simulink library "DABLib"  (R2016b)
settings: Solver=VariableStepAuto  StartTime=0.0  StopTime=10.0  RelTol=1e-3
undefined symbols (not defined in the file or in its folder): ln, sgn
libraries: DABLib x53, simulink_extras x2, simulink x1
(part 1 of 3)
settings Model: Creator=davidlaredorazo  LastModifiedBy=davidlaredorazo
settings DataIOCC: SaveFormat=Array  SignalLoggingSaveFormat=ModelDataLogs
settings OptimizationCC: BlockReduction=off  BooleanDataType=off
settings DebuggingCC: SaveWithParameterizedLinksMsg=none  UnderspecifiedInitializationDetection=Classic  MergeDetectMultiDrivingBlocksExec=none  SignalResolutionControl=TryResolveAllWithWarning  MultiTaskDSMMsg=warning  MultiTaskCondExecSysMsg=none  StrictBusMsg=None
settings HardwareCC: TargetUnknown=on
settings ModelReferenceCC: PropagateSignalLabelsOutOfModel=off

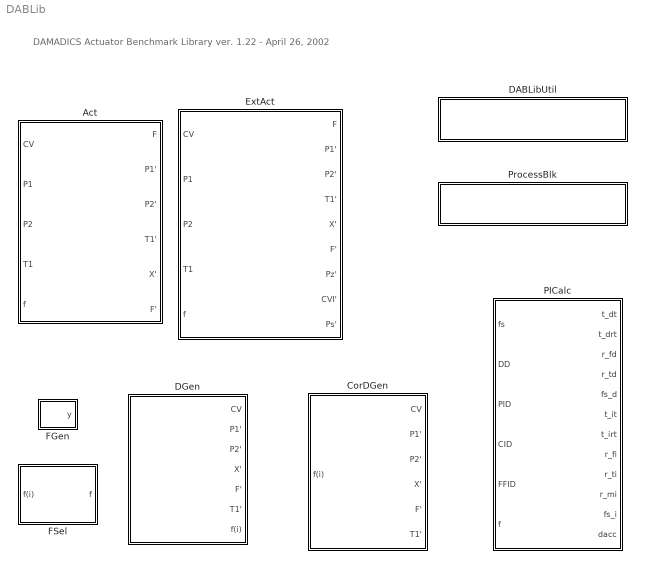
== system DABLib ==
  note: DAMADICS Actuator Benchmark Library ver. 1.22 - April 26, 2002
  Act : Subsystem  mask(Actuator){Dist=off}
      mask prompts: Dist "Disable noise"
      mask help:
      | Actuator 'Act' block is a core of a 'DABLib' library. This block is a model of final control element consisting of positioner, pneumatic motor, control valve and bypass valve.
      | This block reflects the virtual actuator however the parameters of the model were tuned using experimental data achieved during the laboratory tests of: positioner A785, servo-motor type 37 and equalpercentage control valve installed in steam boiler control loop.
      mask Help: web( [ 'file:///' which('DABLib.pdf')]);
      mask Display:
      | plot( [0.2 0.45], [0.3 0.3] )
      | plot( [0.75 0.8], [0.3 0.3] )
      | plot( [0.75 0.75 0.45 0.45 0.75], [0.1 0.5 0.1 0.5 0.1] )
      | plot( [0.6 0.6], [0.3 0.6])
      | plot( [0.45 0.75 0.70 0.5 0.45], [0.6 0.6 0.7 0.7 0.6] )
      | plot( [0.25 0.35 0.35 0.45], [0.9 0.7 0.75 0.55] )
      | text(0.4, 0.9, 'f')
  CorDGen : Subsystem  mask(Benchmark data generator){FSel=NO FAULT}
      mask prompts: FSel "Fault selector:"
      mask help: Data generator 'HIDGen' is a block allowing the generation of data sets with hidden faults for benchmark purposes.
      mask Help: web( [ 'file:///' which('DABLib.pdf')]);
      mask TypeOptions FSel: f1 - Valve clogging | f2 - Valve plug or valve seat sedimentation | f3 - Valve plug or valve seat erosion | f4 - Increased of valve or bushing friction | f5 - External leakage | f6 - Internal leakage | f7 - Medium evaporation or critical flow | f8 - Twisted servo-motor's piston rod | f9 - Servo-motor's housing or terminals tightness | f10 - Servo-motor's diaphragm perforation | f11 - Servo-motor's spring fault | f12 - Electro-pneumatic transducer fault | f13 - Rod displacement sensor fault | f14 - Pressure sensor fault | f15 - Positioner feedback fault | f16 - Positioner supply pressure drop | f17 - Unexpected pressure change across the valve | f18 - Fully or partly opened bypass valves | f19 - Flow rate sensor fault | NO FAULT
      mask Display: fprintf( 'Benchmark Data\n with Hidden Fault\n Generator' )
  DABLibUtil : Subsystem
      mask Display: fprintf(['DABLib Utilities'])
  DGen : Subsystem  mask(Benchmark data generator){FSel=NO FAULT, FType=Abrupt - Small}
      mask prompts: FSel "Fault selector:"; FType "Failure mode:"
      mask help:
      | Data generator 'DGen'  is a block allowing the generation of repeatable patterns of data sets for benchmark purposes.
      |
      | Attention!
      | Not all combinations of parameters are allowed for benchmark. In the case of wrong selection the simulation will be stopped.
      mask init:
      | DSim=0;
      | FSD=1;
      | FFrom = 900;
      | FTo = inf;
      | if FType==4
      |     FMFS=1;
      |     switch FSel
      |         case {2, 3, 5, 6, 9, 11, 18}
      |             FFDT = 3600*24;
      |         case {4, 17}
      |             FFDT = 3600;
      |         case {13}
      |             FFDT = 60*15;
      |         case {20}
      |             FFDT = 0;
      |         otherwise,
      |             FSel = 20;
      |             FFDT = 0;
      |             DSim=1;
      |             warning('Error! - Fault with selected type not specified for benchmark purpose.')
      |     end
      | else
      |     FMFS=0.25*FType;
      |     FFDT=0;
      |     switch FSel
      |         case {3, 4, 5, 6, 9}
      |             DSim=1;
      |             warning('Error! - Fault with selected type not specified for benchmark purpose.')
      |         case {2, 11, 15, 17}
      |             if FType<3
      |                 DSim=1;
      |                 warning('Error! - Fault with selected type not specified for benchmark purpose.')
      |             end
      |         otherwise,
      |     end
      | end
      | switch FSel
      |     case {12, 14, 19}
      |         FSD = -1;
      |     otherwise,
      | end
      mask Help: web( [ 'file:///' which('DABLib.pdf')]);
      mask TypeOptions FSel: f1 - Valve clogging | f2 - Valve plug or valve seat sedimentation | f3 - Valve plug or valve seat erosion | f4 - Increased of valve or bushing friction | f5 - External leakage | f6 - Internal leakage | f7 - Medium evaporation or critical flow | f8 - Twisted servo-motor's piston rod | f9 - Servo-motor's housing or terminals tightness | f10 - Servo-motor's diaphragm perforation | f11 - Servo-motor's spring fault | f12 - Electro-pneumatic transducer fault | f13 - Rod displacement sensor fault | f14 - Pressure sensor fault | f15 - Positioner feedback fault | f16 - Positioner supply pressure drop | f17 - Unexpected pressure change across the valve | f18 - Fully or partly opened bypass valves | f19 - Flow rate sensor fault | NO FAULT
      mask TypeOptions FType: Abrupt - Small | Abrupt - Medium | Abrupt - Large | Incipient
      mask Display: fprintf( 'Benchmark \n Data Generator' )
  ExtAct : Subsystem  mask(Extended Actuator){Dist=on}
      mask prompts: Dist "Disable noise / Analog Transmission"
      mask help:
      | This block is a model of final control element consisting of positioner, pneumatic motor, control valve and bypass valve.
      | This block reflects the virtual actuator however the parameters of the model were tuned using experimental data achieved during the laboratory tests of: positioner A785, servo-motor type 37 and equalpercentage control valve installed in steam boiler control loop.
      mask Help: web( [ 'file:///' which('DABLib.pdf')]);
      mask Display:
      | plot( [0.2 0.45], [0.3 0.3] )
      | plot( [0.75 0.8], [0.3 0.3] )
      | plot( [0.75 0.75 0.45 0.45 0.75], [0.1 0.5 0.1 0.5 0.1] )
      | plot( [0.6 0.6], [0.3 0.6])
      | plot( [0.45 0.75 0.70 0.5 0.45], [0.6 0.6 0.7 0.7 0.6] )
      | plot( [0.25 0.35 0.35 0.45], [0.85 0.7 0.75 0.55] )
      | text(0.4, 0.9, 'f')
      | text(0.2, 1.05, '<<< Extended >>>')
      | text(0.01, 0.03, 'Only for extended researches')
  FGen : Subsystem  mask(Fault generator){From=300, To=inf, MFS=0.5, FDT=0, FSD=1}
      mask prompts: MFS "Max Fault Strength:"; FDT "Fault Development Time:"; FSD "Direction:"
      mask help:
      | Used for generation of abrupt and incipient standarised fault strength values.
      |
      | Parameters:
      | From - fault start time [s]
      | To - fault decay time [s]
      | Max Fault Strength - maximum fault strength value that will be reached during simulation [standarised range - 0 1]
      | Fault Development Time - after this time Max Fault Strength will be reached [s]
      | Direction - defines the sign of fault strength.
      mask init:
      | if FDT==0
      |  FDS = 99999999999999999999999999;
      | else
      |  FDS = MFS / FDT;
      | end
      | if To==inf
      |  To = 99999999999999999999999999;
      | end
      | if FSD >= 0
      | FSD=1;
      | else
      | FSD=-1;
      | end
      mask Help: web( [ 'file:///' which('DABLib.pdf')]);
      mask Display: disp('FGen')
  FSel : Subsystem  mask(Fault vector element attribution){FSel=NO FAULT}
      mask prompts: FSel "Fault selector"
      mask help:
      | Attributes input value to i-th element of the output fault strength vector. The size of the fault strength vector is 19. The values of other output vector elements are set to 0.
      | If 'NO FAULT' option is selected than the fault vector with all 0 elements is produced.
      mask Help: web( [ 'file:///' which('DABLib.pdf')]);
      mask TypeOptions FSel: f1 - Valve clogging | f2 - Valve plug or valve seat sedimentation | f3 - Valve plug or valve seat erosion | f4 - Increased of valve or bushing friction | f5 - External leakage | f6 - Internal leakage | f7 - Medium evaporation or critical flow | f8 - Twisted servo-motor's piston rod | f9 - Servo-motor's housing or terminals tightness | f10 - Servo-motor's diaphragm perforation | f11 - Servo-motor's spring fault | f12 - Electro-pneumatic transducer fault | f13 - Rod displacement sensor fault | f14 - Pressure sensor fault | f15 - Positioner feedback fault | f16 - Positioner supply pressure drop | f17 - Unexpected pressure change across the valve | f18 - Fully or partly opened bypass valves | f19 - Flow rate sensor fault | NO FAULT
      mask Display:
      | text(0.5, 0.75, 'f(i)')
      | plot( [0.5 0.5], [0.7 0.3] )
      | plot( [0.45 0.5 0.55], [0.4 0.3 0.4])
      | text(0.35, 0.1, '[ f(i)   ]')
  PICalc : Subsystem  mask(Performance Indexes Calculator){Step=Other, FSel=NO FAULT, FType=Abrupt - Small, t_on_ini=0, t_hor_ini=100}
      mask prompts: Step "Benchmark:"; FSel "Fault selector:"; FType "Failure mode:"; t_on_ini "Start of Benchmark Zone:"; t_hor_ini "End of Benchmark Zone:"
      mask init:
      | DSim = 0;
      | switch Step
      | 	case {1}
      |       t_on = 300;
      |       if FType==4
      |     		switch FSel
      |         		case {2, 3, 5, 6, 9, 11, 18}
      |             	t_hor = 85500;
      |         		case {4, 17}
      |             	t_hor = 5100;
      |         		case {13}
      |             	t_hor = 2400;
      |         		otherwise,
      |             	t_on = 0;
      |             	t_hor = 0;
      | 					DSim = 1;
      |             	warning('Error! - Fault with selected type not specified for benchmark purpose.')
      |     		end
      | 		else
      | 			t_hor = 1500;
      | 			switch FSel
      |         		case {3, 4, 5, 6, 9}
      |             	t_on = 0;
      |             	t_hor = 0;
      | 					DSim = 1;
      |             	warning('Error! - Fault with selected type not specified for benchmark purpose.')
      |         		case {2, 11, 15, 17}
      |             	if FType<3
      | 	            	t_on = 0;
      |    	         	t_hor = 0;
      | 						DSim = 1;
      |                   warning('Error! - Fault with selected type not specified for benchmark purpose.')
      |                end
      |         		otherwise,
      |     		end
      |       end
      |    case {2}
      | 	            	t_on = 0;
      |    	         	t_hor = 0;
      | 						DSim = 1;
      |                   warning('Not done yet!')
      | 	case {3}
      | 	            	t_on = 0;
      |    	         	t_hor = 0;
      | 						DSim = 1;
      |                   warning('Not done yet!')
      |    otherwise,
      |       t_on = t_on_ini;
      |       t_hor = t_hor_ini;
      | end
      mask TypeOptions Step: I Step | II Step | III Step | Other
      mask TypeOptions FSel: f1 - Valve clogging | f2 - Valve plug or valve seat sedimentation | f3 - Valve plug or valve seat erosion | f4 - Increased of valve or bushing friction | f5 - External leakage | f6 - Internal leakage | f7 - Medium evaporation or critical flow | f8 - Twisted servo-motor's piston rod | f9 - Servo-motor's housing or terminals tightness | f10 - Servo-motor's diaphragm perforation | f11 - Servo-motor's spring fault | f12 - Electro-pneumatic transducer fault | f13 - Rod displacement sensor fault | f14 - Pressure sensor fault | f15 - Positioner feedback fault | f16 - Positioner supply pressure drop | f17 - Unexpected pressure change across the valve | f18 - Fully or partly opened bypass valves | f19 - Flow rate sensor fault | NO FAULT
      mask TypeOptions FType: Abrupt - Small | Abrupt - Medium | Abrupt - Large | Incipient
      mask Display: fprintf( 'Performance\n Indexes\n Calculator' )
  ProcessBlk : Subsystem
      mask Display: fprintf(['Process Components'])

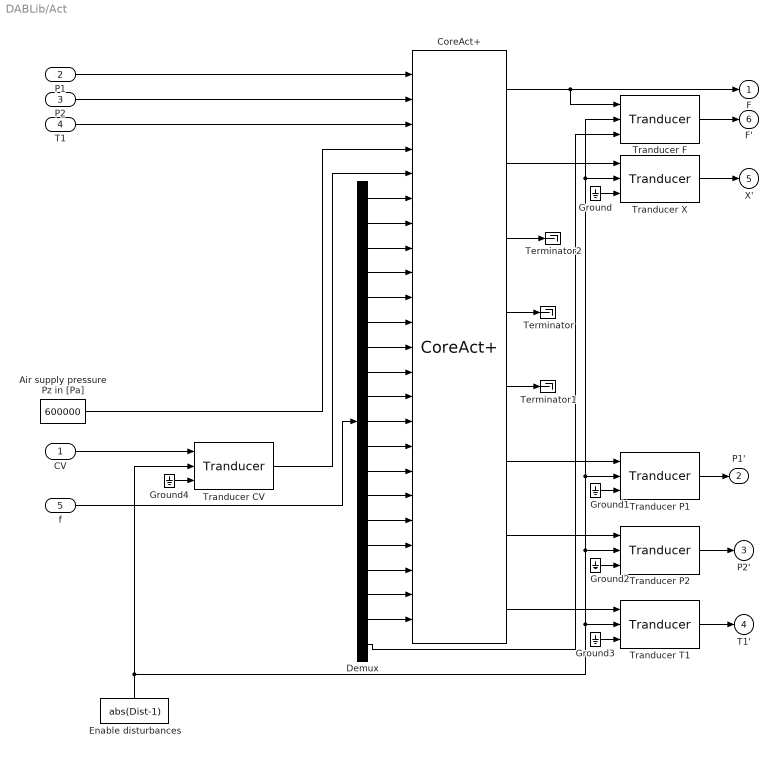
== system DABLib/Act ==
  CV : Inport
  P1 : Inport  Port=2
  P2 : Inport  Port=3
  T1 : Inport  Port=4
  f : Inport  Port=5
  Air supply pressure Pz in [Pa] : Constant  Value=600000
  CoreAct+ : DABLib/DABLibUtil/CoreAct+
  Demux : Demux  Outputs=19
  Enable disturbances : Constant  Value=abs(Dist-1)
  Ground{,1..4} (5 alike) : Ground
  Terminator : Terminator
  Terminator1 : Terminator
  Terminator2 : Terminator
  Tranducer CV : DABLib/DABLibUtil/Tranducer  ScFact=1  Sd=[435435431]
  Tranducer F : DABLib/DABLibUtil/Tranducer  ScFact=40  Sd=[324125]
  Tranducer P1 : DABLib/DABLibUtil/Tranducer  ScFact=4000000  Sd=[123465]
  Tranducer P2 : DABLib/DABLibUtil/Tranducer  ScFact=4000000  Sd=[143534565]
  Tranducer T1 : DABLib/DABLibUtil/Tranducer  ScFact=200  Sd=[452543]
  Tranducer X : DABLib/DABLibUtil/Tranducer  ScFact=1  Sd=[43543513]
  F : Outport  InitialOutput=0
  P1' : Outport  Port=2  InitialOutput=0
  P2' : Outport  Port=3  InitialOutput=0
  T1' : Outport  Port=4  InitialOutput=0
  X' : Outport  Port=5  InitialOutput=0
  F' : Outport  Port=6  InitialOutput=0
  wires:
  CoreAct+/3 -> Terminator2/1
  CoreAct+/4 -> Terminator/1
  CoreAct+/5 -> Terminator1/1
  CoreAct+/1 -> F/1, Tranducer F/1
  f/1 -> Demux/1
  CV/1 -> Tranducer CV/1
  Tranducer CV/1 -> CoreAct+/5
  Demux/1 -> CoreAct+/6
  Demux/2 -> CoreAct+/7
  Demux/3 -> CoreAct+/8
  Demux/4 -> CoreAct+/9
  Demux/5 -> CoreAct+/10
  Demux/6 -> CoreAct+/11
  Demux/7 -> CoreAct+/12
  Demux/8 -> CoreAct+/13
  Demux/9 -> CoreAct+/14
  Demux/10 -> CoreAct+/15
  Demux/11 -> CoreAct+/16
  Demux/12 -> CoreAct+/17
  Demux/13 -> CoreAct+/18
  Demux/14 -> CoreAct+/19
  Demux/15 -> CoreAct+/20
  Demux/16 -> CoreAct+/21
  Demux/17 -> CoreAct+/22
  Demux/18 -> CoreAct+/23
  Enable disturbances/1 -> Tranducer P1/2, Tranducer F/2, Tranducer X/2, Tranducer T1/2, Tranducer P2/2, Tranducer CV/2
  Air supply pressure Pz in [Pa]/1 -> CoreAct+/4
  P1/1 -> CoreAct+/1
  P2/1 -> CoreAct+/2
  Ground4/1 -> Tranducer CV/3
  T1/1 -> CoreAct+/3
  CoreAct+/2 -> Tranducer X/1
  Demux/19 -> Tranducer F/3
  Tranducer X/1 -> X'/1
  Tranducer F/1 -> F'/1
  CoreAct+/6 -> Tranducer P1/1
  Tranducer P1/1 -> P1'/1
  Ground1/1 -> Tranducer P1/3
  CoreAct+/7 -> Tranducer P2/1
  Tranducer P2/1 -> P2'/1
  Ground2/1 -> Tranducer P2/3
  Ground3/1 -> Tranducer T1/3
  Tranducer T1/1 -> T1'/1
  CoreAct+/8 -> Tranducer T1/1
  Ground/1 -> Tranducer X/3

== system DABLib/CorDGen ==
  f(i) : Inport
  Act : DABLib/Act  Dist=off
  Demux : Demux  Outputs=7
  FSel : DABLib/FSel  FSel=NO FAULT
  F_CV3 : Subsystem  mask(Sinus generator){A=0.25, f=0.01, c=0.5}
      mask prompts: A "Amplitude:"; f "Frequency:"; c "Constant component:"
      mask help: y= Asin( 2*3.14ft ) + const
      mask Help: web( [ 'file:///' which('wutalib.html')]);
      mask Display: disp('Sin-gen')
  F_CV4 : Subsystem  mask(Sinus generator){A=175000, f=0.1, c=3500000}
      mask prompts: A "Amplitude:"; f "Frequency:"; c "Constant component:"
      mask help: y= Asin( 2*3.14ft ) + const
      mask Help: web( [ 'file:///' which('wutalib.html')]);
      mask Display: disp('Sin-gen')
  F_CV5 : Subsystem  mask(Sinus generator){A=26000, f=1/pi, c=2600000}
      mask prompts: A "Amplitude:"; f "Frequency:"; c "Constant component:"
      mask help: y= Asin( 2*3.14ft ) + const
      mask Help: web( [ 'file:///' which('wutalib.html')]);
      mask Display: disp('Sin-gen')
  Mux1 : Mux  Inputs=7
  Terminator : Terminator
  "Water temperature [C] " : Constant  Value=43
  Zero-Order Hold : ZeroOrderHold
  CV : Outport  InitialOutput=0
  P1' : Outport  Port=2  InitialOutput=0
  P2' : Outport  Port=3  InitialOutput=0
  X' : Outport  Port=4  InitialOutput=0
  F' : Outport  Port=5  InitialOutput=0
  T1' : Outport  Port=6  InitialOutput=0
  wires:
  "Water temperature [C] "/1 -> Act/4
  FSel/1 -> Act/5
  Act/2 -> Mux1/3
  Act/3 -> Mux1/4
  Act/4 -> Mux1/5
  Act/5 -> Mux1/6
  Act/6 -> Mux1/7
  F_CV3/1(y) -> Act/1, Mux1/1
  Demux/1 -> CV/1
  Demux/2 -> Terminator/1
  Demux/3 -> P1'/1
  Demux/4 -> P2'/1
  Demux/5 -> T1'/1
  Demux/6 -> X'/1
  Demux/7 -> F'/1
  F_CV5/1(y) -> Act/3
  Mux1/1 -> Zero-Order Hold/1
  Zero-Order Hold/1 -> Demux/1
  F_CV4/1(y) -> Act/2
  Act/1 -> Mux1/2
  f(i)/1 -> FSel/1

== system DABLib/DABLibUtil ==
  -1 Correction : Subsystem
  0 Proof Division with -1 correction : Subsystem
  "0, t-t1>0, t2 or 0" : Subsystem
  ADist : Subsystem  mask(Artificial Disturbances){Sine=on, BLWN=on, Seed=[3525342532], ST=0.0025}
      mask prompts: Sine "Sine Enable:"; BLWN "BLWN Enable:"; ST "Sampling Time:"
      mask help: This block introduces artificial generated noise - disturbance.
      mask Help: web( [ 'file:///' which('DABLin.pdf')]);
      mask Display:
      | plot( [0.25 0.5 0.5], [0.25 0.25 0.65] )
      | plot( [0.45 0.5 0.55], [0.6 0.65 0.6])
      | plot( [0.25 0.5 0.51 0.55 0.59 0.61 0.65 0.68 0.7 0.75 0.78 0.8], [0.75 0.75 0.78 0.73 0.8 0.62 0.79 0.6 0.85 0.70 0.8 0.6] )
  ByVal : Subsystem  mask(Valve){}
      mask help: Internal library bloks - not for common use !!
      mask Help: web( [ 'file:///' which('DABLib.pdf')]);
      mask Display: fprintf( 'Bypass \n Valve' )
  Bypass valve opened or bypass valve leaky f18 : Subsystem
  CoreAct : Subsystem  mask(Actuator){}
      mask help: Internal library bloks - not for common use !!
      mask Help: web( [ 'file:///' which('DABLib.pdf')]);
      mask Display: fprintf( 'Core \n Actuator' )
  CoreAct+ : Subsystem  mask(Actuator){}
      mask help: Internal library bloks - not for common use !!
      mask Help: web( [ 'file:///' which('DABLib.pdf')]);
      mask Display: fprintf( 'Core \n Actuator \n + \n Bypass \n Valve \n + \n Ext. Faults' )
  Det or Iso : Subsystem
  Medium evaporation fault f7 : Subsystem
  "Medium evaporation fault f7 " : DABLib/DABLibUtil/Medium evaporation fault f7
  NFSel : Subsystem  mask(Fault vector element selection){FSel=NO FAULT}
      mask prompts: FSel "Fault selector"
      mask help:
      | Attributes i-th element of the input fault strength vector to output value. The size of the fault strength vector is 19.
      | If 'NO FAULT' option is selected than the 0 value is produced.
      mask Help: web( [ 'file:///' which('DABLib.pdf')]);
      mask TypeOptions FSel: f1 - Valve clogging | f2 - Valve plug or valve seat sedimentation | f3 - Valve plug or valve seat erosion | f4 - Increased of valve or bushing friction | f5 - External leakage | f6 - Internal leakage | f7 - Medium evaporation or critical flow | f8 - Twisted servo-motor's piston rod | f9 - Servo-motor's housing or terminals tightness | f10 - Servo-motor's diaphragm perforation | f11 - Servo-motor's spring fault | f12 - Electro-pneumatic transducer fault | f13 - Rod displacement sensor fault | f14 - Pressure sensor fault | f15 - Positioner feedback fault | f16 - Positioner supply pressure drop | f17 - Unexpected pressure change across the valve | f18 - Fully or partly opened bypass valves | f19 - Flow rate sensor fault | NO FAULT
      mask Display:
      | text(0.5, 0.1, 'f(i)')
      | plot( [0.5 0.5], [0.7 0.3] )
      | plot( [0.45 0.5 0.55], [0.4 0.3 0.4])
      | text(0.35, 0.75, '[ f(i)   ]')
  Positioner pressure supply fault f16 : Subsystem
  Tranducer : Subsystem  mask(Sensor){ScFact=1, Sd=[546547567568]}
      mask prompts: ScFact "Scalling Factor:"; Sd "Seed:"
  Treshold2 : Subsystem  mask(Decimal to Binary Conversion){TH=0.5}
      mask prompts: TH "Threshold:"
      mask Display: fprintf( 'Dec \n 2 \n Bin' )

== system DABLib/DGen ==
  Act : DABLib/Act  Dist=off
  Demux : Demux  Outputs=7
  Disable simulation : Constant  Value=DSim
  FGen : DABLib/FGen  From=FFrom  To=FTo  MFS=FMFS  FDT=FFDT  FSD=FSD
  F_CV3 : Subsystem  mask(Sinus generator){A=0.25, f=0.01, c=0.5}
      mask prompts: A "Amplitude:"; f "Frequency:"; c "Constant component:"
      mask help: y= Asin( 2*3.14ft ) + const
      mask Help: web( [ 'file:///' which('wutalib.html')]);
      mask Display: disp('Sin-gen')
  F_CV4 : Subsystem  mask(Sinus generator){A=175000, f=0.1, c=3500000}
      mask prompts: A "Amplitude:"; f "Frequency:"; c "Constant component:"
      mask help: y= Asin( 2*3.14ft ) + const
      mask Help: web( [ 'file:///' which('wutalib.html')]);
      mask Display: disp('Sin-gen')
  F_CV5 : Subsystem  mask(Sinus generator){A=26000, f=1/pi, c=2600000}
      mask prompts: A "Amplitude:"; f "Frequency:"; c "Constant component:"
      mask help: y= Asin( 2*3.14ft ) + const
      mask Help: web( [ 'file:///' which('wutalib.html')]);
      mask Display: disp('Sin-gen')
  Fault Selector : Subsystem
  Mux1 : Mux  Inputs=7
  Stop Simulation : Stop
  Terminator : Terminator
  "Water temperature [C] " : Constant  Value=43
  Zero-Order Hold : ZeroOrderHold
  CV : Outport  InitialOutput=0
  P1' : Outport  Port=2  InitialOutput=0
  P2' : Outport  Port=3  InitialOutput=0
  X' : Outport  Port=4  InitialOutput=0
  F' : Outport  Port=5  InitialOutput=0
  T1' : Outport  Port=6  InitialOutput=0
  f(i) : Outport  Port=7  InitialOutput=0
  wires:
  "Water temperature [C] "/1 -> Act/4
  Fault Selector/1(f(i)) -> Act/5
  Act/2 -> Mux1/3
  Act/3 -> Mux1/4
  Act/4 -> Mux1/5
  Act/5 -> Mux1/6
  Act/6 -> Mux1/7
  F_CV3/1(y) -> Act/1, Mux1/1
  Demux/1 -> CV/1
  Demux/2 -> Terminator/1
  Demux/3 -> P1'/1
  Demux/4 -> P2'/1
  Demux/5 -> T1'/1
  Demux/6 -> X'/1
  Demux/7 -> F'/1
  F_CV5/1(y) -> Act/3
  Disable simulation/1 -> Stop Simulation/1
  FGen/1 -> Fault Selector/1(f)
  Fault Selector/2(max(f)) -> f(i)/1
  Mux1/1 -> Zero-Order Hold/1
  Zero-Order Hold/1 -> Demux/1
  F_CV4/1(y) -> Act/2
  Act/1 -> Mux1/2

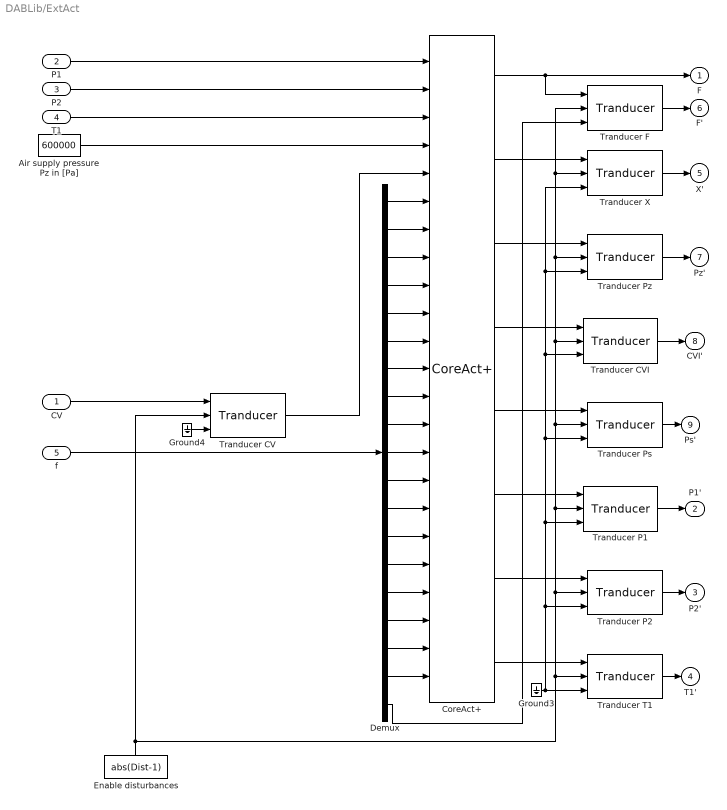
== system DABLib/ExtAct ==
  CV : Inport
  P1 : Inport  Port=2
  P2 : Inport  Port=3
  T1 : Inport  Port=4
  f : Inport  Port=5
  Air supply pressure Pz in [Pa] : Constant  Value=600000
  CoreAct+ : DABLib/DABLibUtil/CoreAct+
  Demux : Demux  Outputs=19
  Enable disturbances : Constant  Value=abs(Dist-1)
  Ground3 : Ground
  Ground4 : Ground
  Tranducer CV : DABLib/DABLibUtil/Tranducer  ScFact=1  Sd=[435435431]
  Tranducer CVI : DABLib/DABLibUtil/Tranducer  ScFact=1  Sd=[647658748]
  Tranducer F : DABLib/DABLibUtil/Tranducer  ScFact=40  Sd=[324125]
  Tranducer P1 : DABLib/DABLibUtil/Tranducer  ScFact=4000000  Sd=[123465]
  Tranducer P2 : DABLib/DABLibUtil/Tranducer  ScFact=4000000  Sd=[143534565]
  Tranducer Ps : DABLib/DABLibUtil/Tranducer  ScFact=1  Sd=[5465462]
  Tranducer Pz : DABLib/DABLibUtil/Tranducer  ScFact=1  Sd=[65487986798]
  Tranducer T1 : DABLib/DABLibUtil/Tranducer  ScFact=200  Sd=[452543]
  Tranducer X : DABLib/DABLibUtil/Tranducer  ScFact=1  Sd=[43543513]
  F : Outport  InitialOutput=0
  P1' : Outport  Port=2  InitialOutput=0
  P2' : Outport  Port=3  InitialOutput=0
  T1' : Outport  Port=4  InitialOutput=0
  X' : Outport  Port=5  InitialOutput=0
  F' : Outport  Port=6  InitialOutput=0
  Pz' : Outport  Port=7  InitialOutput=0
  CVI' : Outport  Port=8  InitialOutput=0
  Ps' : Outport  Port=9  InitialOutput=0
  wires:
  f/1 -> Demux/1
  CV/1 -> Tranducer CV/1
  Enable disturbances/1 -> Tranducer CV/2, Tranducer P2/2, Tranducer P1/2, Tranducer Pz/2, Tranducer X/2, Tranducer F/2, Tranducer CVI/2, Tranducer Ps/2, Tranducer T1/2
  Demux/4 -> CoreAct+/9
  Demux/5 -> CoreAct+/10
  Demux/7 -> CoreAct+/12
  Demux/9 -> CoreAct+/14
  Demux/10 -> CoreAct+/15
  Demux/12 -> CoreAct+/17
  Demux/14 -> CoreAct+/19
  Demux/15 -> CoreAct+/20
  Demux/16 -> CoreAct+/21
  Demux/17 -> CoreAct+/22
  Demux/18 -> CoreAct+/23
  P1/1 -> CoreAct+/1
  CoreAct+/4 -> Tranducer CVI/1
  CoreAct+/6 -> Tranducer P1/1
  Demux/19 -> Tranducer F/3
  Ground4/1 -> Tranducer CV/3
  P2/1 -> CoreAct+/2
  Air supply pressure Pz in [Pa]/1 -> CoreAct+/4
  Tranducer CV/1 -> CoreAct+/5
  Demux/1 -> CoreAct+/6
  Demux/2 -> CoreAct+/7
  Demux/3 -> CoreAct+/8
  Demux/6 -> CoreAct+/11
  Demux/8 -> CoreAct+/13
  Demux/11 -> CoreAct+/16
  Demux/13 -> CoreAct+/18
  CoreAct+/1 -> F/1, Tranducer F/1
  CoreAct+/2 -> Tranducer X/1
  T1/1 -> CoreAct+/3
  Tranducer F/1 -> F'/1
  Tranducer X/1 -> X'/1
  CoreAct+/3 -> Tranducer Pz/1
  Tranducer Pz/1 -> Pz'/1
  Tranducer CVI/1 -> CVI'/1
  CoreAct+/5 -> Tranducer Ps/1
  Tranducer Ps/1 -> Ps'/1
  Tranducer P1/1 -> P1'/1
  CoreAct+/7 -> Tranducer P2/1
  Tranducer P2/1 -> P2'/1
  Tranducer T1/1 -> T1'/1
  CoreAct+/8 -> Tranducer T1/1
  Ground3/1 -> Tranducer T1/3, Tranducer P2/3, Tranducer P1/3, Tranducer Ps/3, Tranducer CVI/3, Tranducer Pz/3, Tranducer X/3

== system DABLib/FGen ==
  Constant5 : Constant  Value=FSD
  Product1 : Product  Inputs=3  SaturateOnIntegerOverflow=on  RndMeth=Zero  InputSameDT=on  OutDataTypeStr=Inherit: Same as first input
  Ramp : Subsystem  mask(Ramp){slope=FDS, start=From, X0=0}
      mask prompts: start "Start time:"; X0 "Initial output:"
      mask help: ramp
      mask Display: plot([0:10],[1,1,1,1:8])
  Saturation8 : Saturate  UpperLimit=MFS  LowerLimit=0
  Step : Step  Time=To  Before=1  After=0
  y : Outport  InitialOutput=0
  wires:
  Ramp/1(out1) -> Saturation8/1
  Saturation8/1 -> Product1/1
  Step/1 -> Product1/2
  Product1/1 -> y/1
  Constant5/1 -> Product1/3

== system DABLib/FSel ==
  f(i) : Inport
  Constant3 : Constant  Value=[1 2 3 4 5 6 7 8 9 10 11 12 13 14 15 16 17 18 19]
  Constant4 : Constant  Value=FSel
  Product : Product  SaturateOnIntegerOverflow=on  RndMeth=Zero  InputSameDT=on  OutDataTypeStr=Inherit: Same as first input
  Relational Operator : RelationalOperator  Operator===  RndMeth=Nearest  InputSameDT=on
  f : Outport  InitialOutput=0
  wires:
  Constant3/1 -> Relational Operator/1
  Constant4/1 -> Relational Operator/2
  Relational Operator/1 -> Product/1
  Product/1 -> f/1
  f(i)/1 -> Product/2

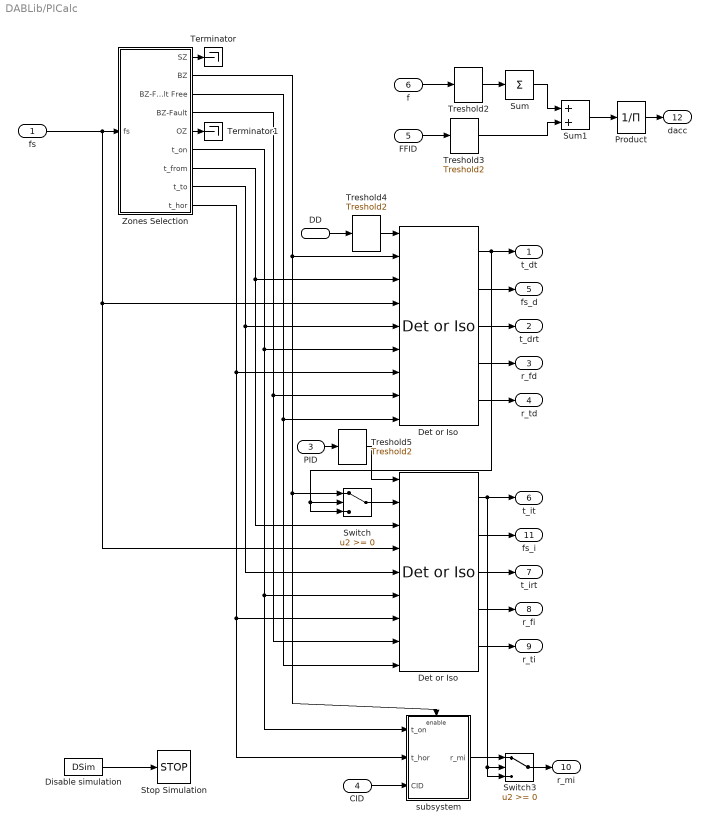
== system DABLib/PICalc ==
  fs : Inport
  DD : Inport  Port=2
  PID : Inport  Port=3
  CID : Inport  Port=4
  FFID : Inport  Port=5
  f : Inport  Port=6
  Det or Iso : DABLib/DABLibUtil/Det or Iso
  "Det or Iso " : DABLib/DABLibUtil/Det or Iso
  Disable simulation : Constant  Value=DSim
  Product : Product  Inputs=/  SaturateOnIntegerOverflow=on  RndMeth=Zero  InputSameDT=on  OutDataTypeStr=Inherit: Same as first input
  Stop Simulation : Stop
  Sum : Sum  Inputs=1  SaturateOnIntegerOverflow=on  InputSameDT=on  OutDataTypeStr=Inherit: Same as first input
  Sum1 : Sum  Inputs=2  SaturateOnIntegerOverflow=on  InputSameDT=on  OutDataTypeStr=Inherit: Same as first input
  Switch : Switch  SaturateOnIntegerOverflow=on  InputSameDT=on
  Switch3 : Switch  SaturateOnIntegerOverflow=on  InputSameDT=on
  Terminator : Terminator
  Terminator1 : Terminator
  Treshold{2..5} (4 alike) : DABLib/DABLibUtil/Treshold2  TH=0.5
  Zones Selection : Subsystem
  subsystem : Subsystem
  t_dt : Outport  InitialOutput=0
  t_drt : Outport  Port=2  InitialOutput=0
  r_fd : Outport  Port=3  InitialOutput=0
  r_td : Outport  Port=4  InitialOutput=0
  fs_d : Outport  Port=5  InitialOutput=0
  t_it : Outport  Port=6  InitialOutput=0
  t_irt : Outport  Port=7  InitialOutput=0
  r_fi : Outport  Port=8  InitialOutput=0
  r_ti : Outport  Port=9  InitialOutput=0
  r_mi : Outport  Port=10  InitialOutput=0
  fs_i : Outport  Port=11  InitialOutput=0
  dacc : Outport  Port=12  InitialOutput=0
  wires:
  Treshold5/1 -> "Det or Iso "/1
  Zones Selection/9("t_hor  ") -> Det or Iso/7, "Det or Iso "/7, subsystem/2(t_hor)
  Zones Selection/8(t_to) -> Det or Iso/5, "Det or Iso "/5
  Zones Selection/7(t_from) -> Det or Iso/3, "Det or Iso "/3
  Zones Selection/6(t_on) -> Det or Iso/6, "Det or Iso "/6, subsystem/1(t_on)
  Zones Selection/2(BZ) -> Det or Iso/2, subsystem/Enable, Switch/1
  Zones Selection/3(BZ-Fault Free) -> Det or Iso/9, "Det or Iso "/9
  fs/1 -> Zones Selection/1(fs), Det or Iso/4, "Det or Iso "/4
  Zones Selection/1(SZ) -> Terminator/1
  Zones Selection/5(OZ) -> Terminator1/1
  Treshold4/1 -> Det or Iso/1
  "Det or Iso "/2 -> fs_i/1
  "Det or Iso "/3 -> t_irt/1
  "Det or Iso "/4 -> r_fi/1
  "Det or Iso "/5 -> r_ti/1
  PID/1 -> Treshold5/1
  DD/1 -> Treshold4/1
  CID/1 -> subsystem/3(CID)
  f/1 -> Treshold2/1
  Treshold2/1 -> Sum/1
  FFID/1 -> Treshold3/1
  Sum/1 -> Sum1/1
  Treshold3/1 -> Sum1/2
  Sum1/1 -> Product/1
  Product/1 -> dacc/1
  Det or Iso/2 -> fs_d/1
  Det or Iso/3 -> t_drt/1
  Det or Iso/4 -> r_fd/1
  Det or Iso/5 -> r_td/1
  subsystem/1(r_mi) -> Switch3/1
  Switch3/1 -> r_mi/1
  "Det or Iso "/1 -> t_it/1, Switch3/2, Switch3/3
  Disable simulation/1 -> Stop Simulation/1
  Switch/1 -> "Det or Iso "/2
  Det or Iso/1 -> t_dt/1, Switch/2, Switch/3
  Zones Selection/4(BZ-Fault) -> Det or Iso/8, "Det or Iso "/8

== system DABLib/ProcessBlk ==
  ProcAct : Subsystem  mask(Process Actuator){}
      mask help:
      | This block is a model of final control element consisting of positioner, pneumatic motor and control valve.
      | This block reflects the virtual actuator however the parameters of the model were tuned using experimental data achieved during the laboratory tests of: positioner A785, servo-motor type 37 and equalpercentage control valve installed in steam boiler control loop.
      mask Help: web( [ 'file:///' which('DABLib.pdf')]);
      mask Display:
      | plot( [0.2 0.45], [0.3 0.3] )
      | plot( [0.75 0.8], [0.3 0.3] )
      | plot( [0.75 0.75 0.45 0.45 0.75], [0.1 0.5 0.1 0.5 0.1] )
      | plot( [0.6 0.6], [0.3 0.6])
      | plot( [0.45 0.75 0.70 0.5 0.45], [0.6 0.6 0.7 0.7 0.6] )
      | plot( [0.25 0.35 0.35 0.45], [0.85 0.7 0.75 0.55] )
      | text(0.4, 0.9, 'f')
      | text(0.25, 1.05, '<<< Process >>>')
      | text(0.05, 0.03, 'Only for process connection')
  ProcBV : Subsystem  mask(Process By-pass Valve){}
      mask help: This block is a model of by-pass valve
      mask Help: web( [ 'file:///' which('DABLib.pdf')]);
      mask Display:
      | text(0.25, 1.05, '<<< Process >>>')
      | fprintf( 'Bypass \n Valve' )
      | text(0.05, 0.03, 'Only for process connection')
  ProcTran : Subsystem  mask(Process Transducer){ScFact=1, EN=on, Sd=[546547567568], FSel=NO FAULT}
      mask prompts: ScFact "Scalling Factor:"; EN "Enable disturbances:"; Sd "Seed:"; FSel "Fault selector"
      mask Help: web( [ 'file:///' which('DABLib.pdf')]);
      mask TypeOptions FSel: f1 - Valve clogging | f2 - Valve plug or valve seat sedimentation | f3 - Valve plug or valve seat erosion | f4 - Increased of valve or bushing friction | f5 - External leakage | f6 - Internal leakage | f7 - Medium evaporation or critical flow | f8 - Twisted servo-motor's piston rod | f9 - Servo-motor's housing or terminals tightness | f10 - Servo-motor's diaphragm perforation | f11 - Servo-motor's spring fault | f12 - Electro-pneumatic transducer fault | f13 - Rod displacement sensor fault | f14 - Pressure sensor fault | f15 - Positioner feedback fault | f16 - Positioner supply pressure drop | f17 - Unexpected pressure change across the valve | f18 - Fully or partly opened bypass valves | f19 - Flow rate sensor fault | NO FAULT
      mask Display: text(0.5, 0.5, 'T')
  Proc_f16 : Subsystem  mask(Fault){}
      mask Help: web( [ 'file:///' which('DABLib.pdf')]);
      mask Display:
      | plot( [0.3 0.4 0.4 0.5], [0.85 0.4 0.65 0.25] )
      | text(0.4, 0.9, 'f7')
  Proc_f18 : Subsystem  mask(Fault){}
      mask Help: web( [ 'file:///' which('DABLib.pdf')]);
      mask Display:
      | plot( [0.3 0.4 0.4 0.5], [0.85 0.4 0.65 0.25] )
      | text(0.4, 0.9, 'f7')
  Proc_f7 : Subsystem  mask(Fault){}
      mask Help: web( [ 'file:///' which('DABLib.pdf')]);
      mask Display:
      | plot( [0.3 0.4 0.4 0.5], [0.85 0.4 0.65 0.25] )
      | text(0.4, 0.9, 'f7')

== system DABLib/CorDGen/F_CV3 ==
  P6 : Constant  Value=c
  Signal Generator : SignalGenerator  Amplitude=A  Frequency=f
  suma : Sum  SaturateOnIntegerOverflow=on  InputSameDT=on  OutDataTypeStr=Inherit: Same as first input
  y : Outport  InitialOutput=0
  wires:
  Signal Generator/1 -> suma/1
  P6/1 -> suma/2
  suma/1 -> y/1

== system DABLib/CorDGen/F_CV4 ==
  P6 : Constant  Value=c
  Signal Generator : SignalGenerator  Amplitude=A  Frequency=f
  suma : Sum  SaturateOnIntegerOverflow=on  InputSameDT=on  OutDataTypeStr=Inherit: Same as first input
  y : Outport  InitialOutput=0
  wires:
  Signal Generator/1 -> suma/1
  P6/1 -> suma/2
  suma/1 -> y/1

== system DABLib/CorDGen/F_CV5 ==
  P6 : Constant  Value=c
  Signal Generator : SignalGenerator  Amplitude=A  Frequency=f
  suma : Sum  SaturateOnIntegerOverflow=on  InputSameDT=on  OutDataTypeStr=Inherit: Same as first input
  y : Outport  InitialOutput=0
  wires:
  Signal Generator/1 -> suma/1
  P6/1 -> suma/2
  suma/1 -> y/1

== system DABLib/DABLibUtil/-1 Correction ==
  In : Inport
  Clock : Clock
  Relational Operator : RelationalOperator  Operator=<=  RndMeth=Nearest  InputSameDT=on
  Switch : Switch  Threshold=0.5  SaturateOnIntegerOverflow=on  InputSameDT=on
  "const  " : Constant  Value=-1
  out : Outport  InitialOutput=0
  wires:
  Switch/1 -> out/1
  In/1 -> Switch/1, Relational Operator/1
  Relational Operator/1 -> Switch/2
  "const  "/1 -> Switch/3
  Clock/1 -> Relational Operator/2

== system DABLib/DABLibUtil/0 Proof Division with -1 correction ==
  Denominator : Inport
  Numerator : Inport  Port=2
  Product : Product  Inputs=/*  SaturateOnIntegerOverflow=on  RndMeth=Zero  InputSameDT=on  OutDataTypeStr=Inherit: Same as first input
  Relational Operator : RelationalOperator  Operator=>  RndMeth=Nearest  InputSameDT=on
  Switch1 : Switch  Threshold=1  SaturateOnIntegerOverflow=on  InputSameDT=on
  Switch2 : Switch  Threshold=1  SaturateOnIntegerOverflow=on  InputSameDT=on
  const  1 : Constant  Value=0
  const  2 : Constant  Value=-1
  const  3 : Constant  Value=-1
  Division : Outport  InitialOutput=0
  wires:
  const  1/1 -> Relational Operator/2
  Product/1 -> Switch1/1
  Numerator/1 -> Product/2
  Switch1/1 -> Division/1
  const  2/1 -> Switch1/3
  Denominator/1 -> Relational Operator/1, Switch2/1
  Switch2/1 -> Product/1
  const  3/1 -> Switch2/3
  Relational Operator/1 -> Switch1/2, Switch2/2

== system DABLib/DABLibUtil/0, t-t1>0, t2 or 0 ==
  t_2 : Inport
  t_1 : Inport  Port=2
  Clock : Clock
  Relational Operator : RelationalOperator  Operator=>  RndMeth=Nearest  InputSameDT=on
  Sum : Sum  Inputs=+-  SaturateOnIntegerOverflow=on  InputSameDT=on  OutDataTypeStr=Inherit: Same as first input
  Switch : Switch  Threshold=-0.5  SaturateOnIntegerOverflow=on  InputSameDT=on
  Switch1 : Switch  Threshold=1  SaturateOnIntegerOverflow=on  InputSameDT=on
  Switch2 : Switch  Threshold=-0.5  SaturateOnIntegerOverflow=on  InputSameDT=on
  "const  " : Constant  Value=0
  const  1 : Constant  Value=0
  const  2 : Constant  Value=0
  dt : Outport  InitialOutput=0
  wires:
  "const  "/1 -> Switch1/3
  t_1/1 -> Switch2/2, Sum/2
  t_2/1 -> Switch/1, Switch/2
  Clock/1 -> Switch/3
  Switch/1 -> Sum/1
  const  1/1 -> Relational Operator/2
  Relational Operator/1 -> Switch1/2
  const  2/1 -> Switch2/3
  Switch2/1 -> dt/1
  Switch1/1 -> Switch2/1
  Sum/1 -> Relational Operator/1, Switch1/1

== system DABLib/DABLibUtil/ADist ==
  x : Inport
  EN : Inport  Port=2
  BLWN : Constant  Value=BLWN+1
  Band-Limited White Noise : simulink/Sources/Band-Limited White Noise  Cov=[0.0025*2/1000000]  Ts=ST  seed=Seed
  Constant : Constant  Value=0
  Constant1 : Constant  Value=0
  Multiport Switch : MultiPortSwitch  Inputs=2  SaturateOnIntegerOverflow=on  InputSameDT=on
  Multiport Switch1 : MultiPortSwitch  Inputs=2  SaturateOnIntegerOverflow=on  InputSameDT=on
  Multiport Switch2 : MultiPortSwitch  Inputs=2  SaturateOnIntegerOverflow=on  InputSameDT=on
  Sine : Constant  Value=Sine+1
  Sine1 : Constant
  Sinus Generator : SignalGenerator  Amplitude=0.0025  Frequency=50
  Sum : Sum  Inputs=+++  SaturateOnIntegerOverflow=on  InputSameDT=on  OutDataTypeStr=Inherit: Same as first input
  Sum1 : Sum  SaturateOnIntegerOverflow=on  InputSameDT=on  OutDataTypeStr=Inherit: Same as first input
  y : Outport  InitialOutput=0
  wires:
  Sine1/1 -> Sum1/2
  Sum1/1 -> Multiport Switch2/1
  EN/1 -> Sum1/1
  Multiport Switch2/1 -> y/1
  Sum/1 -> Multiport Switch2/3
  x/1 -> Multiport Switch2/2, Sum/1
  Multiport Switch/1 -> Sum/2
  Sine/1 -> Multiport Switch/1
  Sinus Generator/1 -> Multiport Switch/3
  Constant/1 -> Multiport Switch/2
  BLWN/1 -> Multiport Switch1/1
  Band-Limited White Noise/1 -> Multiport Switch1/3
  Constant1/1 -> Multiport Switch1/2
  Multiport Switch1/1 -> Sum/3

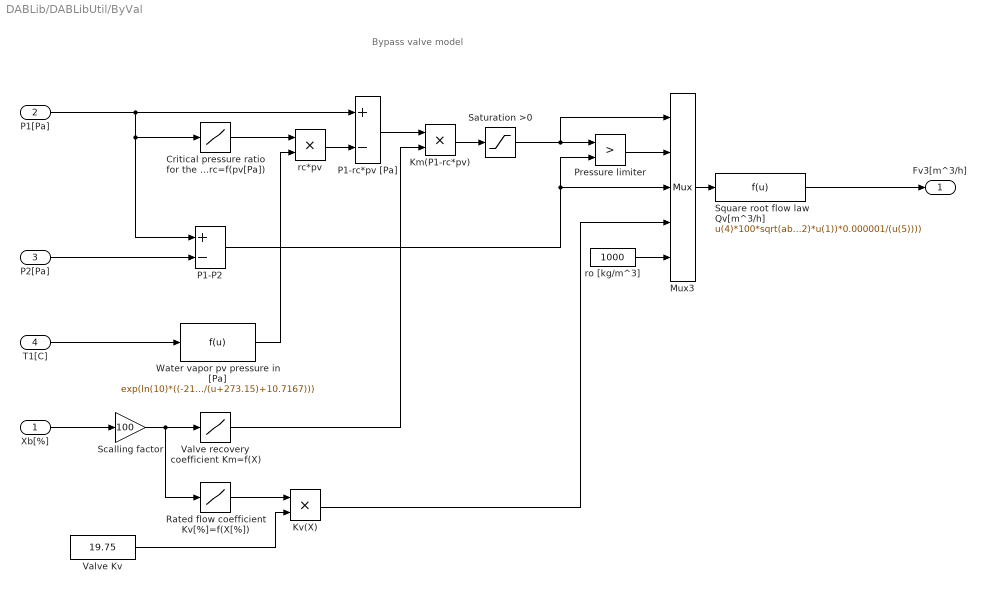
== system DABLib/DABLibUtil/ByVal ==
  note: Bypass valve model
  Xb[%] : Inport
  P1[Pa] : Inport  Port=2
  P2[Pa] : Inport  Port=3
  T1[C] : Inport  Port=4
  "Critical pressure ratio for the water rc=f(pv[Pa]) " : Lookup  InputValues="[0  1723763 3447527 6895055 13790111 17237639 20685166]"  Table=[0.94 0.87 0.84 0.79 0.75 0.725 0.685]  SaturateOnIntegerOverflow=on
  Km(P1-rc*pv) : Product  SaturateOnIntegerOverflow=on  RndMeth=Zero  InputSameDT=on  OutDataTypeStr=Inherit: Same as first input
  Kv(X) : Product  SaturateOnIntegerOverflow=on  RndMeth=Zero  InputSameDT=on  OutDataTypeStr=Inherit: Same as first input
  Mux3 : Mux  Inputs=5
  P1-P2 : Sum  Inputs=+-  SaturateOnIntegerOverflow=on  InputSameDT=on  OutDataTypeStr=Inherit: Same as first input
  P1-rc*pv [Pa] : Sum  Inputs=+-  SaturateOnIntegerOverflow=on  InputSameDT=on  OutDataTypeStr=Inherit: Same as first input
  Pressure limiter : RelationalOperator  Operator=>  RndMeth=Nearest  InputSameDT=on
  Rated flow coefficient Kv[%]=f(X[%]) : Lookup  InputValues=[0 10 20 30 40 50 60 70 80 90 100]  Table=[1.0 0.9 0.8 0.7 0.6 0.5 0.4 0.3 0.2 0.1 0.0]  SaturateOnIntegerOverflow=on
  Saturation >0 : Saturate  UpperLimit=inf  LowerLimit=0
  Scalling factor : Gain  Gain=100  SaturateOnIntegerOverflow=on  OutDataTypeStr=Inherit: Same as input  ParamDataTypeStr=Inherit: Same as input
  Square root flow law Qv[m^3/h] : Fcn  Expr=u(4)*100*sqrt(abs((u(2)*u(3)+!u(2)*u(1))*0.000001/(u(5))))
  Valve Kv : Constant  Value=19.75
  Valve recovery coefficient Km=f(X) : Lookup  InputValues=[0 10 20 30 40 50 60 70 80 90 100]  Table="[0.45  0.5 0.555 0.61 0.67 0.725 0.785 0.85 0.90 0.95 1.00]"  SaturateOnIntegerOverflow=on
  Water vapor pv pressure in [Pa] : Fcn  Expr=exp(ln(10)*((-2141/(u+273.15)+10.7167)))
  rc*pv : Product  SaturateOnIntegerOverflow=on  RndMeth=Zero  InputSameDT=on  OutDataTypeStr=Inherit: Same as first input
  ro [kg/m^3] : Constant  Value=1000
  Fv3[m^3/h] : Outport
  wires:
  Valve recovery coefficient Km=f(X)/1 -> Km(P1-rc*pv)/2
  P1-P2/1 -> Mux3/3, Pressure limiter/2
  Water vapor pv pressure in [Pa]/1 -> rc*pv/2
  Scalling factor/1 -> Rated flow coefficient Kv[%]=f(X[%])/1, Valve recovery coefficient Km=f(X)/1
  Xb[%]/1 -> Scalling factor/1
  Kv(X)/1 -> Mux3/4
  P1[Pa]/1 -> P1-rc*pv [Pa]/1, P1-P2/1, "Critical pressure ratio for the water rc=f(pv[Pa]) "/1
  Saturation >0/1 -> Pressure limiter/1, Mux3/1
  Pressure limiter/1 -> Mux3/2
  rc*pv/1 -> P1-rc*pv [Pa]/2
  P1-rc*pv [Pa]/1 -> Km(P1-rc*pv)/1
  Km(P1-rc*pv)/1 -> Saturation >0/1
  "Critical pressure ratio for the water rc=f(pv[Pa]) "/1 -> rc*pv/1
  Square root flow law Qv[m^3/h]/1 -> Fv3[m^3/h]/1
  Mux3/1 -> Square root flow law Qv[m^3/h]/1
  Valve Kv/1 -> Kv(X)/2
  Rated flow coefficient Kv[%]=f(X[%])/1 -> Kv(X)/1
  P2[Pa]/1 -> P1-P2/2
  ro [kg/m^3]/1 -> Mux3/5
  T1[C]/1 -> Water vapor pv pressure in [Pa]/1

== system DABLib/DABLibUtil/Bypass valve opened or bypass valve leaky f18 ==
  note: Fault  f18 entry
      | Bypass open or external leakage or leaky valve fault
  f18<0,1> : Inport
  " " : Fcn  Expr=(1-u(1)*u(2))
  Fault range in [%] <0..1> : Constant  Value=1.0
  "Fault streght saturation " : Saturate  UpperLimit=1.0  LowerLimit=0
  Mux4 : Mux  Inputs=2
  Xb[%] : Outport
  wires:
  Mux4/1 -> " "/1
  f18<0,1>/1 -> "Fault streght saturation "/1
  " "/1 -> Xb[%]/1
  "Fault streght saturation "/1 -> Mux4/2
  Fault range in [%] <0..1>/1 -> Mux4/1

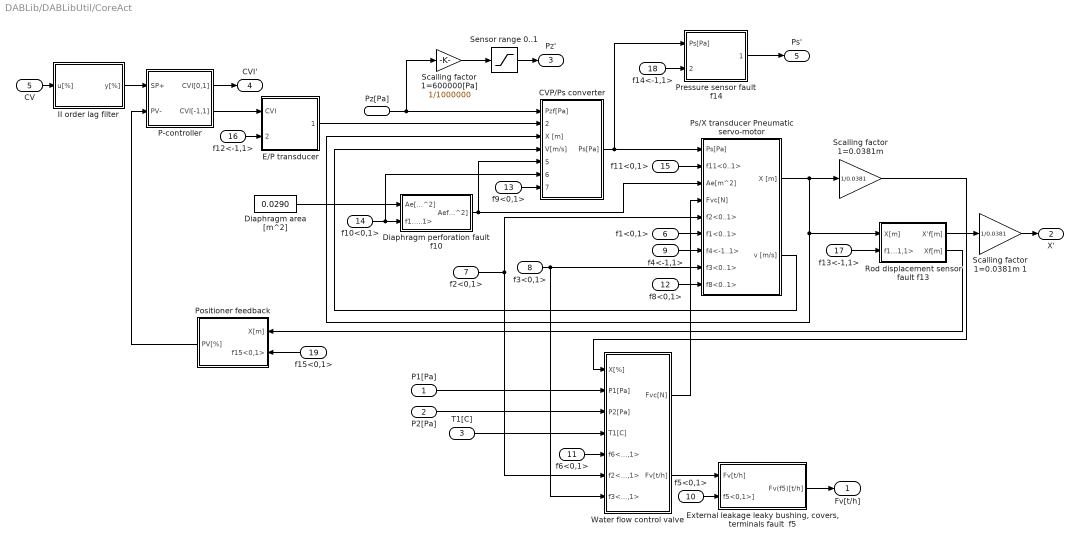
== system DABLib/DABLibUtil/CoreAct ==
  P1[Pa] : Inport
  P2[Pa] : Inport  Port=2
  T1[C] : Inport  Port=3
  Pz[Pa] : Inport  Port=4
  CV : Inport  Port=5
  f1<0,1> : Inport  Port=6
  f2<0,1> : Inport  Port=7
  f3<0,1> : Inport  Port=8
  f4<-1,1> : Inport  Port=9
  f5<0,1> : Inport  Port=10
  f6<0,1> : Inport  Port=11
  f8<0,1> : Inport  Port=12
  f9<0,1> : Inport  Port=13
  f10<0,1> : Inport  Port=14
  f11<0,1> : Inport  Port=15
  f12<-1,1> : Inport  Port=16
  f13<-1,1> : Inport  Port=17
  f14<-1,1> : Inport  Port=18
  f15<0,1> : Inport  Port=19
  "  E/P transducer" : Subsystem
  CVP/Ps converter : Subsystem
  Diaphragm perforation fault f10 : Subsystem
  Diaphragm area [m^2] : Constant  Value=0.0290
  "External leakage leaky bushing, covers, terminals fault  f5" : Subsystem
  II order lag filter : Subsystem
  P-controller : Subsystem
  Positioner feedback : Subsystem
  Pressure sensor fault f14 : Subsystem
  Ps/X transducer Pneumatic servo-motor : Subsystem
  Rod displacement sensor fault f13 : Subsystem
  "Scalling factor 1=0.0381m " : Gain  Gain=1/0.0381  SaturateOnIntegerOverflow=on  OutDataTypeStr=Inherit: Same as input  ParamDataTypeStr=Inherit: Same as input
  Scalling factor 1=0.0381m 1 : Gain  Gain=1/0.0381  SaturateOnIntegerOverflow=on  OutDataTypeStr=Inherit: Same as input  ParamDataTypeStr=Inherit: Same as input
  Scalling factor 1=600000[Pa] : Gain  Gain=1/1000000  SaturateOnIntegerOverflow=on  OutDataTypeStr=Inherit: Same as input  ParamDataTypeStr=Inherit: Same as input
  Sensor range 0..1 : Saturate  UpperLimit=1  LowerLimit=0
  Water flow control valve : Subsystem
  Fv[t/h] : Outport  InitialOutput=0
  X' : Outport  Port=2  InitialOutput=0
  Pz' : Outport  Port=3  InitialOutput=0
  CVI' : Outport  Port=4  InitialOutput=0
  Ps' : Outport  Port=5  InitialOutput=0
  wires:
  P2[Pa]/1 -> Water flow control valve/3(P2[Pa])
  P1[Pa]/1 -> Water flow control valve/2(P1[Pa])
  "External leakage leaky bushing, covers, terminals fault  f5"/1(Fv(f5)[t/h]) -> Fv[t/h]/1
  CVP/Ps converter/1(Ps[Pa]) -> Pressure sensor fault f14/1(Ps[Pa]), Ps/X transducer Pneumatic servo-motor/1(Ps[Pa])
  f14<-1,1>/1 -> Pressure sensor fault f14/2(f14<-1,1>])
  Scalling factor 1=0.0381m 1/1 -> X'/1
  P-controller/1(CVI[0,1]) -> CVI'/1
  P-controller/2(CVI[-1,1]) -> "  E/P transducer"/1(CVI)
  f12<-1,1>/1 -> "  E/P transducer"/2(f12<-1,1>)
  Positioner feedback/1(PV[%]) -> P-controller/2(PV-)
  Water flow control valve/1(Fvc[N]) -> Ps/X transducer Pneumatic servo-motor/4(Fvc[N])
  "Scalling factor 1=0.0381m "/1 -> Water flow control valve/1(X[%])
  Water flow control valve/2(Fv[t/h]) -> "External leakage leaky bushing, covers, terminals fault  f5"/1(Fv[t/h])
  f6<0,1>/1 -> Water flow control valve/5(f6<0,1>)
  f5<0,1>/1 -> "External leakage leaky bushing, covers, terminals fault  f5"/2(f5<0,1>])
  f11<0,1>/1 -> Ps/X transducer Pneumatic servo-motor/2(f11<0..1>)
  f1<0,1>/1 -> Ps/X transducer Pneumatic servo-motor/6(f1<0..1>)
  f4<-1,1>/1 -> Ps/X transducer Pneumatic servo-motor/7(f4<-1..1>)
  f8<0,1>/1 -> Ps/X transducer Pneumatic servo-motor/9(f8<0..1>)
  Pressure sensor fault f14/1(Psf[0..1]) -> Ps'/1
  Sensor range 0..1/1 -> Pz'/1
  Scalling factor 1=600000[Pa]/1 -> Sensor range 0..1/1
  Pz[Pa]/1 -> Scalling factor 1=600000[Pa]/1, CVP/Ps converter/1(Pzf[Pa])
  II order lag filter/1(y[%]) -> P-controller/1(SP+)
  CV/1 -> II order lag filter/1(u[%])
  Rod displacement sensor fault f13/2(Xf[m]) -> Positioner feedback/1(X[m])
  Rod displacement sensor fault f13/1(X'f[m]) -> Scalling factor 1=0.0381m 1/1
  Diaphragm area [m^2]/1 -> Diaphragm perforation fault f10/1(Ae[m^2])
  Diaphragm perforation fault f10/1(Aef[m^2]) -> CVP/Ps converter/5(Ae [m^2]), Ps/X transducer Pneumatic servo-motor/3(Ae[m^2])
  "  E/P transducer"/1(CVP[%]) -> CVP/Ps converter/2(CVP[%])
  f9<0,1>/1 -> CVP/Ps converter/7(f9<0,1>)
  f15<0,1>/1 -> Positioner feedback/2(f15<0,1>)
  f10<0,1>/1 -> Diaphragm perforation fault f10/2(f10 <0..1>), CVP/Ps converter/6(f10<0,1>)
  Ps/X transducer Pneumatic servo-motor/2(v [m/s]) -> CVP/Ps converter/4(V[m/s])
  Ps/X transducer Pneumatic servo-motor/1(X [m]) -> "Scalling factor 1=0.0381m "/1, Rod displacement sensor fault f13/1(X[m]), CVP/Ps converter/3(X [m])
  f13<-1,1>/1 -> Rod displacement sensor fault f13/2(f13<-1,1>)
  f2<0,1>/1 -> Water flow control valve/6(f2<0,1>), Ps/X transducer Pneumatic servo-motor/5(f2<0..1>)
  f3<0,1>/1 -> Water flow control valve/7(f3<0,1>), Ps/X transducer Pneumatic servo-motor/8(f3<0..1>)
  T1[C]/1 -> Water flow control valve/4(T1[C])

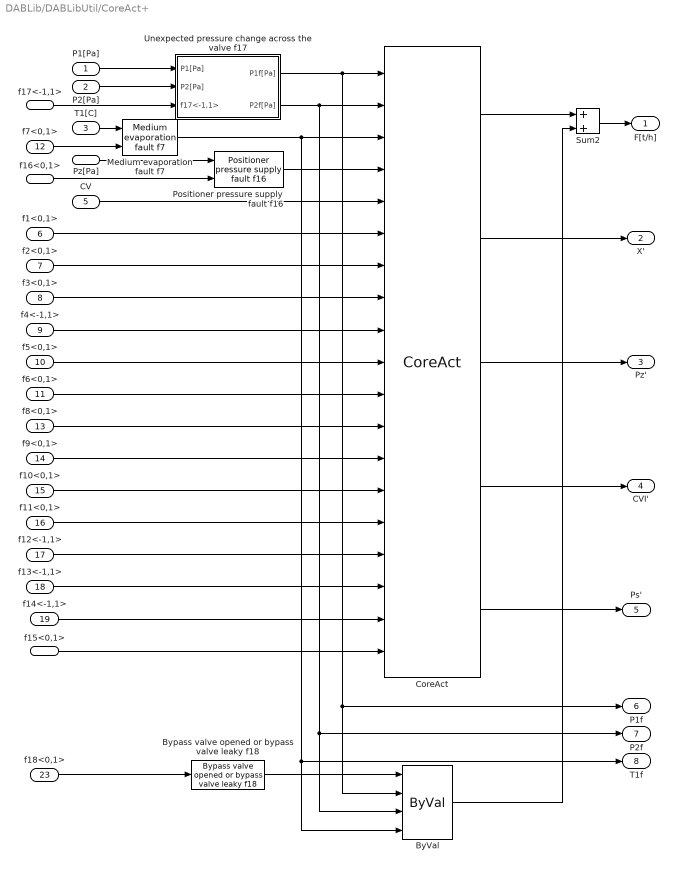
== system DABLib/DABLibUtil/CoreAct+ ==
  P1[Pa] : Inport
  P2[Pa] : Inport  Port=2
  T1[C] : Inport  Port=3
  Pz[Pa] : Inport  Port=4
  CV : Inport  Port=5
  f1<0,1> : Inport  Port=6
  f2<0,1> : Inport  Port=7
  f3<0,1> : Inport  Port=8
  f4<-1,1> : Inport  Port=9
  f5<0,1> : Inport  Port=10
  f6<0,1> : Inport  Port=11
  f7<0,1> : Inport  Port=12
  f8<0,1> : Inport  Port=13
  f9<0,1> : Inport  Port=14
  f10<0,1> : Inport  Port=15
  f11<0,1> : Inport  Port=16
  f12<-1,1> : Inport  Port=17
  f13<-1,1> : Inport  Port=18
  f14<-1,1> : Inport  Port=19
  f15<0,1> : Inport  Port=20
  f16<0,1> : Inport  Port=21
  f17<-1,1> : Inport  Port=22
  f18<0,1> : Inport  Port=23
  ByVal : DABLib/DABLibUtil/ByVal
  Bypass valve opened or bypass valve leaky f18 : DABLib/DABLibUtil/Bypass valve opened  or bypass valve leaky  f18
  CoreAct : DABLib/DABLibUtil/CoreAct
  "Medium evaporation fault f7 " : DABLib/DABLibUtil/Medium evaporation fault f7
  Positioner pressure supply fault f16 : DABLib/DABLibUtil/Positioner pressure  supply fault f16
  Sum2 : Sum  SaturateOnIntegerOverflow=on  InputSameDT=on  OutDataTypeStr=Inherit: Same as first input
  Unexpected pressure change across the valve f17 : Subsystem
  F[t/h] : Outport  InitialOutput=0
  X' : Outport  Port=2  InitialOutput=0
  Pz' : Outport  Port=3  InitialOutput=0
  CVI' : Outport  Port=4  InitialOutput=0
  Ps' : Outport  Port=5  InitialOutput=0
  P1f : Outport  Port=6  InitialOutput=0
  P2f : Outport  Port=7  InitialOutput=0
  T1f : Outport  Port=8  InitialOutput=0
  wires:
  Bypass valve opened or bypass valve leaky f18/1 -> ByVal/1
  f6<0,1>/1 -> CoreAct/11
  f16<0,1>/1 -> Positioner pressure supply fault f16/2
  f17<-1,1>/1 -> Unexpected pressure change across the valve f17/3(f17<-1,1>)
  Positioner pressure supply fault f16/1 -> CoreAct/4
  Pz[Pa]/1 -> Positioner pressure supply fault f16/1
  f4<-1,1>/1 -> CoreAct/9
  P2[Pa]/1 -> Unexpected pressure change across the valve f17/2(P2[Pa])
  P1[Pa]/1 -> Unexpected pressure change across the valve f17/1(P1[Pa])
  Unexpected pressure change across the valve f17/2(P2f[Pa]) -> ByVal/3, P2f/1, CoreAct/2
  Unexpected pressure change across the valve f17/1(P1f[Pa]) -> ByVal/2, P1f/1, CoreAct/1
  CoreAct/1 -> Sum2/1
  ByVal/1 -> Sum2/2
  CoreAct/3 -> Pz'/1
  CoreAct/2 -> X'/1
  f5<0,1>/1 -> CoreAct/10
  f3<0,1>/1 -> CoreAct/8
  f2<0,1>/1 -> CoreAct/7
  f1<0,1>/1 -> CoreAct/6
  CV/1 -> CoreAct/5
  CoreAct/5 -> Ps'/1
  T1[C]/1 -> "Medium evaporation fault f7 "/1
  f7<0,1>/1 -> "Medium evaporation fault f7 "/2
  "Medium evaporation fault f7 "/1 -> CoreAct/3, ByVal/4, T1f/1
  f18<0,1>/1 -> Bypass valve opened or bypass valve leaky f18/1
  f8<0,1>/1 -> CoreAct/12
  f9<0,1>/1 -> CoreAct/13
  f10<0,1>/1 -> CoreAct/14
  f11<0,1>/1 -> CoreAct/15
  f12<-1,1>/1 -> CoreAct/16
  f13<-1,1>/1 -> CoreAct/17
  f14<-1,1>/1 -> CoreAct/18
  f15<0,1>/1 -> CoreAct/19
  CoreAct/4 -> CVI'/1
  Sum2/1 -> F[t/h]/1

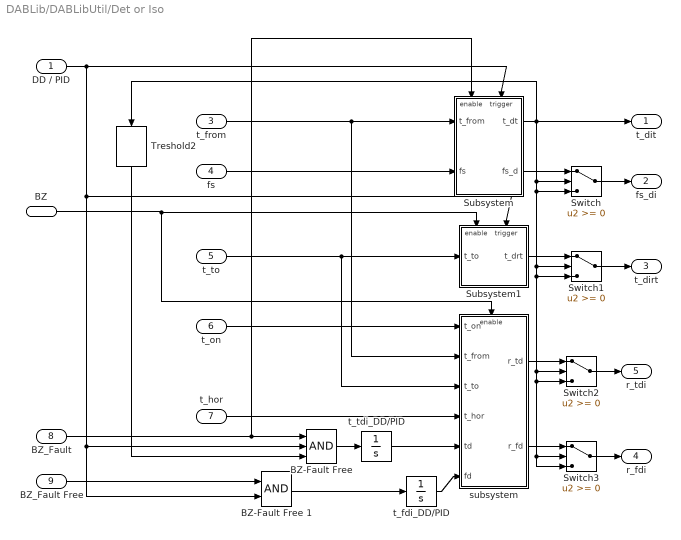
== system DABLib/DABLibUtil/Det or Iso ==
  DD / PID : Inport
  BZ : Inport  Port=2
  t_from : Inport  Port=3
  fs : Inport  Port=4
  t_to : Inport  Port=5
  t_on : Inport  Port=6
  t_hor : Inport  Port=7
  BZ_Fault : Inport  Port=8
  BZ_Fault Free : Inport  Port=9
  "BZ-Fault Free " : Logic  Inputs=3
  BZ-Fault Free 1 : Logic
  Subsystem : Subsystem
  Subsystem1 : Subsystem
  Switch{,1..3} (4 alike) : Switch  SaturateOnIntegerOverflow=on  InputSameDT=on
  Treshold2 : DABLib/DABLibUtil/Treshold2  TH=0.5
  subsystem : Subsystem
  t_fdi_DD/PID : Integrator
  t_tdi_DD/PID : Integrator
  t_dit : Outport  InitialOutput=0
  fs_di : Outport  Port=2  InitialOutput=0
  t_dirt : Outport  Port=3  InitialOutput=0
  r_fdi : Outport  Port=4  InitialOutput=0
  r_tdi : Outport  Port=5  InitialOutput=0
  wires:
  BZ_Fault/1 -> Subsystem/Enable, "BZ-Fault Free "/1
  BZ/1 -> subsystem/Enable, Subsystem1/Enable
  Treshold2/1 -> "BZ-Fault Free "/3
  Switch3/1 -> r_fdi/1
  subsystem/2(r_fd) -> Switch3/1
  Switch2/1 -> r_tdi/1
  subsystem/1(r_td) -> Switch2/1
  Subsystem1/1(t_drt) -> Switch1/1
  Switch1/1 -> t_dirt/1
  Subsystem/1(t_dt) -> Treshold2/1, Switch/3, Switch1/3, Switch3/3, Switch3/2, Switch2/3, Switch2/2, Switch1/2, Switch/2, t_dit/1
  Subsystem/2(fs_d) -> Switch/1
  Switch/1 -> fs_di/1
  t_to/1 -> subsystem/3(t_to), Subsystem1/1(t_to)
  t_from/1 -> subsystem/2(t_from), Subsystem/1(t_from)
  BZ_Fault Free/1 -> BZ-Fault Free 1/1
  t_hor/1 -> subsystem/4(t_hor)
  t_on/1 -> subsystem/1(t_on)
  fs/1 -> Subsystem/2(fs)
  t_tdi_DD/PID/1 -> subsystem/5(td)
  "BZ-Fault Free "/1 -> t_tdi_DD/PID/1
  BZ-Fault Free 1/1 -> t_fdi_DD/PID/1
  t_fdi_DD/PID/1 -> subsystem/6(fd)
  DD / PID/1 -> Subsystem/Trigger, Subsystem1/Trigger, "BZ-Fault Free "/2, BZ-Fault Free 1/2
